simulink model "NES"  (R2019a)
settings: Solver=VariableStepAuto  StartTime=0.0  StopTime=10.0  RelTol=1e-3
InitFcn:
  | init
values from neighbouring files (symbols this model uses):
  c = params.c    [S2dot.m]    (also in cdisp.m; importdata.m = 100; ode45_code.m = 0.01)
  k = params.k    [S2dot.m]    (also in cdisp.m; importdata.m = 20000; main_QuestionE.m = 50000; ode45_code.m = 5)
  m = params.m    [S2dot.m]    (also in importdata.m = 0.005; main_QuestionE.m = 527.1; ode45_code.m = 1)
undefined symbols (not defined in the file or in its folder): amplitude, final_value, frequency, init_value, noise, S, s_initial, sample_time_noise, Sdot, sdot_initial, siggen, stp, stp_time
libraries: simulink x1
settings Model: Creator=NegarPajooh  LastModifiedBy=NegarPajooh

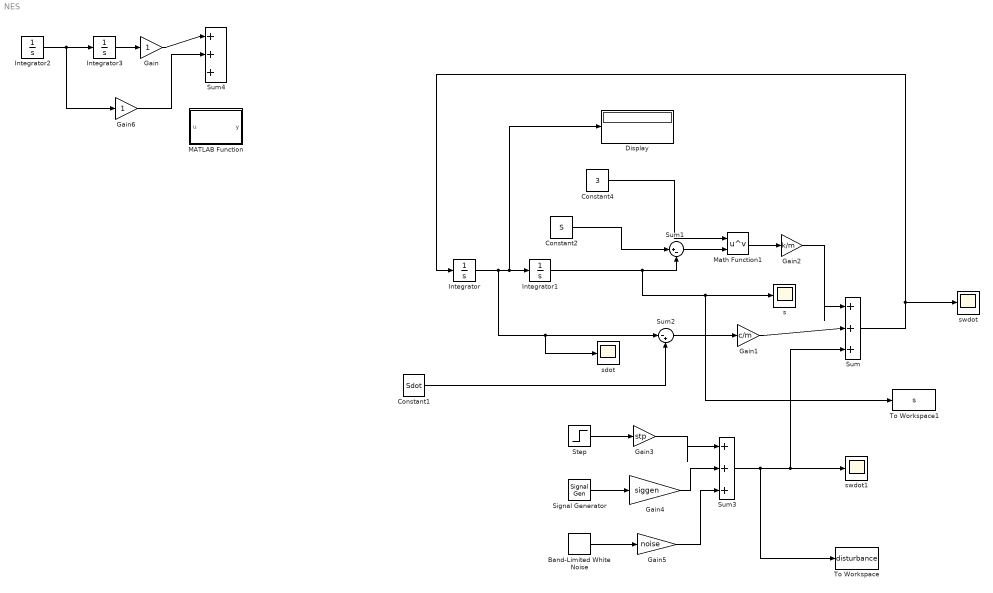
== system NES ==
  Band-Limited White Noise : simulink/Sources/Band-Limited White Noise  Cov=noise_power  Ts=sample_time_noise  seed=seed
  Constant1 : Constant  Value=Sdot
  Constant2 : Constant  Value=S
  Constant4 : Constant  Value=3
  Display : Display
  Gain : Gain
  Gain1 : Gain  Gain=c/m
  Gain2 : Gain  Gain=k/m
  Gain3 : Gain  Gain=stp
  Gain4 : Gain  Gain=siggen
  Gain5 : Gain  Gain=noise
  Gain6 : Gain
  Integrator : Integrator  InitialCondition=sdot_initial
  Integrator1 : Integrator  InitialCondition=s_initial
  Integrator2 : Integrator  InitialCondition=sdot_initial
  Integrator3 : Integrator  InitialCondition=sdot_initial
  MATLAB Function : MATLAB Function  TreatAsAtomicUnit=on
  Math Function1 : Math  Operator=pow  SaturateOnIntegerOverflow=on
  Signal Generator : SignalGenerator  Amplitude=amplitude  Frequency=frequency  Units=rad/sec
  Step : Step  Time=stp_time  Before=init_value  After=final_value  SampleTime=0
  Sum : Sum  Inputs=|+++
  Sum1 : Sum  Inputs=|+-
  Sum2 : Sum  Inputs=|-+
  Sum3 : Sum  Inputs=|+++
  Sum4 : Sum  Inputs=|+++
  To Workspace : ToWorkspace  VariableName=disturbance  SaveFormat=Structure With Time  SampleTime=-1
  To Workspace1 : ToWorkspace  VariableName=s  SaveFormat=Structure With Time  SampleTime=-1
  s : Scope
  sdot : Scope
  swdot : Scope
  swdot1 : Scope
  wires:
  Integrator1/1 -> To Workspace1/1, s/1, Sum1/2
  Integrator/1 -> sdot/1, Sum2/1, Display/1, Integrator1/1
  Sum/1 -> swdot/1, Integrator/1
  Constant1/1 -> Sum2/2
  Constant2/1 -> Sum1/1
  Sum1/1 -> Math Function1/2
  Sum2/1 -> Gain1/1
  Constant4/1 -> Math Function1/1
  Math Function1/1 -> Gain2/1
  Gain2/1 -> Sum/1
  Gain1/1 -> Sum/2
  Sum3/1 -> To Workspace/1, swdot1/1, Sum/3
  Band-Limited White Noise/1 -> Gain5/1
  Signal Generator/1 -> Gain4/1
  Step/1 -> Gain3/1
  Gain5/1 -> Sum3/3
  Gain4/1 -> Sum3/2
  Gain3/1 -> Sum3/1
  Integrator2/1 -> Gain6/1, Integrator3/1
  Gain/1 -> Sum4/1
  Integrator3/1 -> Gain/1
  Gain6/1 -> Sum4/2

== matlab function NES/MATLAB Function ==
  data: u input; y output
function y = fcn(u)

y = u;
